simulink library "UXFD_Lib"  (R2016b)
settings: Solver=ode45  StartTime=0.0  StopTime=10.0  RelTol=1e-3  EnableMultiTasking=on
undefined symbols (not defined in the file): BreakpointData, BreakpointData1, BreakpointData2, BreakpointData_One_A, BreakpointData_Two_A, E2E_P01DataIDMode, E2E_P01ReceiverStatusType, EnumClass, iBit, initalValue, No_Runnable_Period, ObB_EidBsgStDerat_C, p_OVERRIDE_MASTER_SWITCH, SlDemoSign, SwitchOff_P, SwitchOn_P, Table, TableData_M, VCCTi33, VSysD_FidVehDerat1_C
libraries: simulink x28, CCMLib x11, UXFD_Lib x8, canmsglib x2, PTCC_Lib x1, hdlsllib x1
(part 3 of 7)

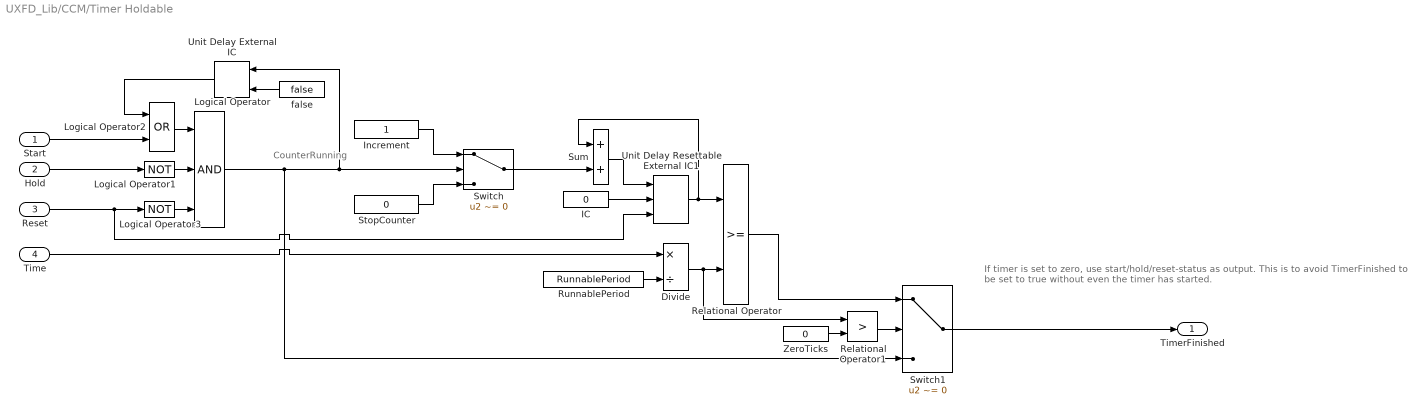
== system UXFD_Lib/CCM/Timer Holdable ==
  note: If timer is set to zero, use start/hold/reset-status as output.
      | This is to avoid TimerFinished to be set to true without even the timer has started.
  note: CounterRunning
  Start : Inport  OutDataTypeStr=boolean
  Hold : Inport  Port=2  OutDataTypeStr=boolean
  Reset : Inport  Port=3  OutDataTypeStr=boolean
  Time : Inport  Port=4  OutDataTypeStr=timeDataType
  Divide : Product  Inputs=*/  OutDataTypeStr=VCCUInt32  RndMeth=Round  SaturateOnIntegerOverflow=on
  IC : Constant  Value=0  OutDataTypeStr=VCCUInt32  SampleTime=-1
  Increment : Constant  OutDataTypeStr=VCCUInt32  SampleTime=-1
  Logical Operator : Logic  Inputs=3  AllPortsSameDT=off  OutDataTypeStr=boolean
  Logical Operator1 : Logic  Operator=NOT  AllPortsSameDT=off  OutDataTypeStr=boolean
  Logical Operator2 : Logic  Operator=OR  AllPortsSameDT=off  OutDataTypeStr=boolean
  Logical Operator3 : Logic  Operator=NOT  AllPortsSameDT=off  OutDataTypeStr=boolean
  Relational Operator : RelationalOperator  OutDataTypeStr=boolean  RndMeth=Nearest
  Relational Operator1 : RelationalOperator  Operator=>  OutDataTypeStr=boolean  RndMeth=Nearest
  RunnablePeriod : Constant  Value=RunnablePeriod  OutDataTypeStr=VCCTiSamplePerd  SampleTime=-1
  StopCounter : Constant  Value=0  OutDataTypeStr=VCCUInt32  SampleTime=-1
  Sum : Sum  OutDataTypeStr=VCCUInt32  SaturateOnIntegerOverflow=on
  Switch : Switch  Criteria=u2 ~= 0  SaturateOnIntegerOverflow=on
  Switch1 : Switch  Criteria=u2 ~= 0  SaturateOnIntegerOverflow=on
  Unit Delay External IC : simulink/Additional Math & Discrete/Additional Discrete/Unit Delay External IC  tsamp=-1
  Unit Delay Resettable External IC1 : CCMLib/Unit Delay Resettable External IC  dataType=VCCUInt32
  ZeroTicks : Constant  Value=0  OutDataTypeStr=VCCUInt32  SampleTime=-1
  false : Constant  Value=false  OutDataTypeStr=boolean  SampleTime=-1
  TimerFinished : Outport  OutDataTypeStr=boolean
  wires:
  Sum/1 -> Unit Delay Resettable External IC1/1
  IC/1 -> Unit Delay Resettable External IC1/2
  Time/1 -> Divide/1
  Reset/1 -> Unit Delay Resettable External IC1/3, Logical Operator3/1
  Logical Operator3/1 -> Logical Operator/3
  Switch1/1 -> TimerFinished/1
  Divide/1 -> Relational Operator1/1, Relational Operator/2
  Relational Operator/1 -> Switch1/1
  Relational Operator1/1 -> Switch1/2
  ZeroTicks/1 -> Relational Operator1/2
  RunnablePeriod/1 -> Divide/2
  StopCounter/1 -> Switch/3
  Increment/1 -> Switch/1
  Switch/1 -> Sum/2
  Unit Delay Resettable External IC1/1 -> Relational Operator/1, Sum/1
  Unit Delay External IC/1 -> Logical Operator2/1
  Start/1 -> Logical Operator2/2
  Logical Operator/1 -> Switch1/3, Unit Delay External IC/1, Switch/2
  false/1 -> Unit Delay External IC/2
  Logical Operator2/1 -> Logical Operator/1
  Hold/1 -> Logical Operator1/1
  Logical Operator1/1 -> Logical Operator/2

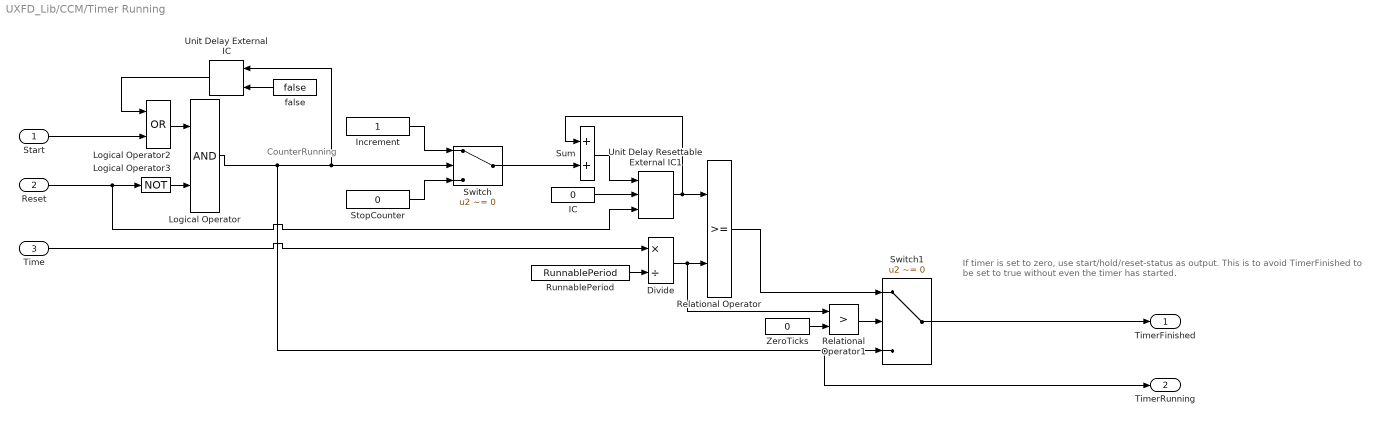
== system UXFD_Lib/CCM/Timer Running ==
  note: If timer is set to zero, use start/hold/reset-status as output.
      | This is to avoid TimerFinished to be set to true without even the timer has started.
  note: CounterRunning
  Start : Inport  OutDataTypeStr=boolean
  Reset : Inport  Port=2  OutDataTypeStr=boolean
  Time : Inport  Port=3  OutDataTypeStr=timeDataType
  Divide : Product  Inputs=*/  OutDataTypeStr=VCCUInt32  RndMeth=Round  SaturateOnIntegerOverflow=on
  IC : Constant  Value=0  OutDataTypeStr=VCCUInt32  SampleTime=-1
  Increment : Constant  OutDataTypeStr=VCCUInt32  SampleTime=-1
  Logical Operator : Logic  AllPortsSameDT=off  OutDataTypeStr=boolean
  Logical Operator2 : Logic  Operator=OR  AllPortsSameDT=off  OutDataTypeStr=boolean
  Logical Operator3 : Logic  Operator=NOT  AllPortsSameDT=off  OutDataTypeStr=boolean
  Relational Operator : RelationalOperator  OutDataTypeStr=boolean  RndMeth=Nearest
  Relational Operator1 : RelationalOperator  Operator=>  OutDataTypeStr=boolean  RndMeth=Nearest
  RunnablePeriod : Constant  Value=RunnablePeriod  OutDataTypeStr=VCCTiSamplePerd  SampleTime=-1
  StopCounter : Constant  Value=0  OutDataTypeStr=VCCUInt32  SampleTime=-1
  Sum : Sum  OutDataTypeStr=VCCUInt32  SaturateOnIntegerOverflow=on
  Switch : Switch  Criteria=u2 ~= 0  SaturateOnIntegerOverflow=on
  Switch1 : Switch  Criteria=u2 ~= 0  SaturateOnIntegerOverflow=on
  Unit Delay External IC : simulink/Additional Math & Discrete/Additional Discrete/Unit Delay External IC  tsamp=-1
  Unit Delay Resettable External IC1 : CCMLib/Unit Delay Resettable External IC  dataType=VCCUInt32
  ZeroTicks : Constant  Value=0  OutDataTypeStr=VCCUInt32  SampleTime=-1
  false : Constant  Value=false  OutDataTypeStr=boolean  SampleTime=-1
  TimerFinished : Outport  OutDataTypeStr=boolean
  TimerRunning : Outport  Port=2  OutDataTypeStr=boolean
  wires:
  Sum/1 -> Unit Delay Resettable External IC1/1
  IC/1 -> Unit Delay Resettable External IC1/2
  Time/1 -> Divide/1
  Reset/1 -> Unit Delay Resettable External IC1/3, Logical Operator3/1
  Logical Operator3/1 -> Logical Operator/2
  Switch1/1 -> TimerFinished/1
  Divide/1 -> Relational Operator1/1, Relational Operator/2
  Relational Operator/1 -> Switch1/1
  Relational Operator1/1 -> Switch1/2
  ZeroTicks/1 -> Relational Operator1/2
  RunnablePeriod/1 -> Divide/2
  StopCounter/1 -> Switch/3
  Increment/1 -> Switch/1
  Switch/1 -> Sum/2
  Unit Delay Resettable External IC1/1 -> Sum/1, Relational Operator/1
  Unit Delay External IC/1 -> Logical Operator2/1
  Start/1 -> Logical Operator2/2
  Logical Operator/1 -> TimerRunning/1, Switch1/3, Unit Delay External IC/1, Switch/2
  false/1 -> Unit Delay External IC/2
  Logical Operator2/1 -> Logical Operator/1

== system UXFD_Lib/CCM/Unit Delay External IC ==
  u : Inport  OutDataTypeStr=dataType
  IC : Inport  Port=2  OutDataTypeStr=dataType
  Constant : Constant  Value=true  OutDataTypeStr=boolean  SampleTime=-1
  Switch : Switch  Criteria=u2 ~= 0  SaturateOnIntegerOverflow=on
  Unit Delay : UnitDelay  InitialCondition=false  SampleTime=-1
      settings: AttributesFormatString=X0=%<X0>
  Unit Delay1 : UnitDelay  SampleTime=-1
      settings: AttributesFormatString=X0=%<X0>
  y : Outport  OutDataTypeStr=dataType
  wires:
  Switch/1 -> y/1
  IC/1 -> Switch/3
  u/1 -> Unit Delay1/1
  Unit Delay1/1 -> Switch/1
  Constant/1 -> Unit Delay/1
  Unit Delay/1 -> Switch/2

== system UXFD_Lib/CCM/Unit Delay Resettable ==
  u : Inport  OutDataTypeStr=dataType
  R : Inport  Port=2  OutDataTypeStr=boolean
  Constant : Constant  Value=false  OutDataTypeStr=boolean  SampleTime=-1
  Logical Operator : Logic  Operator=OR  AllPortsSameDT=off  OutDataTypeStr=boolean
  Logical Operator1 : Logic  Operator=NOT  AllPortsSameDT=off  OutDataTypeStr=boolean
  Switch : Switch  Criteria=u2 ~= 0  SaturateOnIntegerOverflow=on
  Switch1 : Switch  Criteria=u2 ~= 0  SaturateOnIntegerOverflow=on
  Unit Delay : UnitDelay  InitialCondition=true  SampleTime=-1
      settings: AttributesFormatString=X0=%<X0>
  Unit Delay1 : UnitDelay  InitialCondition=initialCondition  SampleTime=-1
      settings: AttributesFormatString=X0=%<X0>
  initialCondition : Constant  Value=initialCondition  OutDataTypeStr=dataType  SampleTime=-1
  y : Outport  OutDataTypeStr=dataType
  wires:
  Constant/1 -> Unit Delay/1
  Switch/1 -> y/1
  Logical Operator/1 -> Switch/2
  Unit Delay/1 -> Logical Operator/2
  R/1 -> Logical Operator/1, Logical Operator1/1
  Logical Operator1/1 -> Switch1/2
  initialCondition/1 -> Switch1/3, Switch/1
  Switch1/1 -> Unit Delay1/1
  Unit Delay1/1 -> Switch/3
  u/1 -> Switch1/1

== system UXFD_Lib/CCM/Unit Delay Resettable External IC ==
  u : Inport  OutDataTypeStr=dataType
  IC : Inport  Port=2  OutDataTypeStr=dataType
  R : Inport  Port=3  OutDataTypeStr=boolean
  Constant : Constant  Value=true  OutDataTypeStr=boolean  SampleTime=-1
  Logical Operator : Logic  Operator=NOT  AllPortsSameDT=off  OutDataTypeStr=boolean
  Logical Operator1 : Logic  AllPortsSameDT=off  OutDataTypeStr=boolean
  Switch : Switch  Criteria=u2 ~= 0  SaturateOnIntegerOverflow=on
  Switch1 : Switch  Criteria=u2 ~= 0  SaturateOnIntegerOverflow=on
  Unit Delay : UnitDelay  InitialCondition=false  SampleTime=-1
      settings: AttributesFormatString=X0=%<X0>
  Unit Delay1 : UnitDelay  SampleTime=-1
      settings: AttributesFormatString=X0=%<X0>
  y : Outport  OutDataTypeStr=dataType
  wires:
  Logical Operator1/1 -> Switch/2
  Unit Delay/1 -> Logical Operator1/1
  Switch1/1 -> Unit Delay1/1
  IC/1 -> Switch/3, Switch1/3
  u/1 -> Switch1/1
  R/1 -> Logical Operator/1
  Logical Operator/1 -> Logical Operator1/2, Switch1/2
  Constant/1 -> Unit Delay/1
  Unit Delay1/1 -> Switch/1
  Switch/1 -> y/1

== system UXFD_Lib/Custom/CAN ==
  note: CAN
  CAN Pack : canmsglib/CAN Pack  MsgList=(none)  MsgName=CAN Msg  MsgIDType=Standard (11-bit identifier)  MsgIdentifier=0  MsgLength=8  NSignals=0  StartBits=0  SignalSizes=0  ByteOrders=0  DataTypes=0  MultiplexTypes=0  MultiplexValues=0  Factors=0  Offsets=0  Minimums=0  Maximums=0  Remote=off
      settings: DataFormat=raw data
  CAN Unpack : canmsglib/CAN Unpack  MsgName=CAN Msg  MsgIDType=Standard (11-bit identifier)  MsgIdentifier=0  MsgLength=8  NSignals=0  IDPort=off  TimestampPort=off  ErrorPort=off  RemotePort=off  LengthPort=off  StatusPort=off  StartBits=0  SignalSizes=0  ByteOrders=0  DataTypes=0  MultiplexTypes=0  MultiplexValues=0  Factors=0  Offsets=0  Minimums=0  Maximums=0
      settings: DataFormat=raw data
  CAN_Receive : Subsystem  mask(CAN Message Receive( GLib TM )){}
      mask help:
      | Input： DataType CAN_Message Signal and handle
      | Output：If Received success , Return Value is 1
      mask Display:
      | port_label('input',1,'Message')
      | port_label('input',2,'Handle')
      | port_label('output',1,'ReturnValue')
      | disp('ACTION_CANBSW_RecMsg_S')
  CAN_Transmit : Subsystem  mask(CAN Message Transmit( GLib TM )){}
      mask help:
      | Input： DataType CAN_Message Signal and handle
      | Output：If Transmited success , Return Value is 1
      mask Display:
      | port_label('input',1,'Message')
      | port_label('input',2,'Handle')
      | port_label('output',1,'ReturnValue')
      | disp('ACTION_CANBSW_SndMsg_S')
  CanHex2Signed : Subsystem  mask(CAN signal Hex2Signed){BitLengthValue=32, FactorValue=0.001, OffsetValue=0}
      mask prompts: BitLengthValue "CAN Signal Bit Length（0<u<=32bit）"; FactorValue "Factor"; OffsetValue "Offset"
      mask help: convert the hex to signed value, please specified bit length of varible in CAN matrix, the maximum bit length in CAN matrixa may be 32bit; Also, please specified the factor and offset, then execute Phy=hex*factor+offset.
      mask init:
      | % The mask parameter returns the one-based index of the selection
      | FactorValue;
      | OffsetValue;
      | BitLengthValue;
      | % To obtain the string corresponding to the selection, use get_param
      | blk = gcb;
      | FactorString = get_param(blk,'FactorValue');
      | OffsetString = get_param(blk,'OffsetValue');
      | BitSzieString = get_param(blk,'BitLengthValue');
      | 
      |     % Convert the string into a single to use the value under the mask
      |     BitLength = single(str2num(BitSzieString)); 
      |     Factor=single(str2num(FactorString)); 
      |     Offset=single(str2num(OffsetString));
      mask Display:
      | fprintf('CAN signal convert\nBitLength: %d\nFactor: %2.4f\nOffset: %2.4f',...
      |     BitLengthValue,FactorValue,OffsetValue);
  Get_MsgLength : Subsystem  mask(Get CAN Message Length( GLib TM )){}
      mask help:
      | Input： DataType CAN_Message Signal
      | Output：CAN Message Length
      mask Display:
      | port_label('input',1,'Message')
      | port_label('output',1,'Length')
      | disp('Msg_Length_S')
  xbackground1 : Subsystem
      mask Display: disp(' ')

== system UXFD_Lib/Custom/Diagnose ==
  note: Diagnose
  Dem_SetEventStatus : Subsystem  mask(SL Blockset Dem_SetEventStatus){EventID=ObB_EidBsgStDerat_C}
      mask prompts: EventID "Dem Event ID"
      mask help:
      | Interface block to call Dem_SetEventStatus.
      | The output of the block can be captured by using Dem_SetEventStatus blocks with the same EventID.
      mask TypeOptions EventID: DEM_EventID/Value
      mask Display:
      | id = get_param(gcb,'EventID');
      | text(0.55,0.9,sprintf('Dem_SetEventStatus\nEventID: %s', id),...
      |     'horizontalAlignment','center',...
      |     'verticalAlignment', 'top');
      | 
      | 
      | port_label('input',1,'EveSt');
      | port_label('input',2,'bEna');
  Fim_GetFunctionPermission : Subsystem  mask(SL Blockset Fim_GetFunctionPermission){FunctionID=VSysD_FidVehDerat1_C}
      mask prompts: FunctionID "FIM FunctionID"
      mask help:
      | Interface block to call Fim_GetFunctionPermission.
      | The output of the block can be stimulated by using Fim_GetFunctionPermission_Stimuli blocks with the same FunctionID.
      mask TypeOptions FunctionID: FIM_EventID/Value
      mask Display:
      | id = get_param(gcb,'FunctionID');
      | text(0.45,0.9,sprintf('Fim_GetFunctionPermission\nFunctionID: %s', id),...
      |     'horizontalAlignment','center',...
      |     'verticalAlignment', 'top');
      | 
      | port_label('output',1,'bEna');
  xbackground1 : Subsystem
      mask Display: disp(' ')

== system UXFD_Lib/Custom/PIN ==
  note: HW PIN
  PIN ADC : Subsystem  mask(PIN ADC){g_functionName=Sws_Io_Adc_Get_xxx, g_getValue=2}
      mask prompts: g_functionName "应用层接口函数"; g_getValue "测试输出返回值"
      mask help:
      | This block is for ASW to get Hardware's  ADC PIN Value
      | Function: uint16 Sws_Io_Adc_Get_xxx(void)
      mask Display: text(0.08,0.67,'Get Pin Analog Input','horizontalAlignment', 'left', 'verticalAlignment', 'top');
  PIN DI : Subsystem  mask(PIN DI){g_functionName=Sws_Io_Dio_Get_xxx, g_getValue=1}
      mask prompts: g_functionName "应用层接口函数"; g_getValue "测试输出返回值"
      mask help:
      | This block is for ASW to get Hardware's  DI PIN Value
      | Function: boolean Sws_Io_Dio_Get_xxx()
      mask Display: text(0.08,0.67,'Get Pin Digital Input','horizontalAlignment', 'left', 'verticalAlignment', 'top');
  PIN DO : Subsystem  mask(PIN DO){g_functionName=Sws_Io_Dio_Set_O_S_xxx}
      mask prompts: g_functionName "应用层接口函数"
      mask help:
      | This block is for ASW to set Hardware's  DO PIN Value
      | Function:  void Sws_Io_Dio_Set_O_S_xxx(boolean stSignal_b)
      mask Display: text(0.08,0.67,'Set Pin Digital Output','horizontalAlignment', 'left', 'verticalAlignment', 'top');
  PIN DO1 : Subsystem  mask(PIN PWMOUT){g_functionName=Sws_Io_PWM_Set_O_S_xxx}
      mask prompts: g_functionName "应用层接口函数"
      mask help:
      | This block is for ASW to set Hardware's  PWM PIN Value
      | Function:  void Sws_Io_PWM_Set_O_S_xxx(sint16 Duty_s16,uint32 Period_u32)
      mask Display: text(0.08,0.67,'Set Pin PWM Output','horizontalAlignment', 'left', 'verticalAlignment', 'top');
  PIN ICU : Subsystem  mask(PIN ICU){g_functionName=Sws_Io_Icu_GetPeriod_xxx, g_getValue=50}
      mask prompts: g_functionName "应用层接口函数"; g_getValue "测试输出返回值"
      mask help:
      | This block is for ASW to get Hardware's  ICU PIN Value
      | Function:  Sws_Io_Icu_GetDutyCyclexxx(void)
      mask Display: text(0.08,0.67,'Get Pin ICU Input','horizontalAlignment', 'left', 'verticalAlignment', 'top');
  xbackground1 : Subsystem
      mask Display: disp(' ')

== system UXFD_Lib/Standard/Bit Operation ==
  Bit Clear : simulink/Logic and Bit Operations/Bit Clear  iBit=0
  Bit Set : simulink/Logic and Bit Operations/Bit Set  iBit=0
  Bit Shift : hdlsllib/HDL Operations/Bit Shift  mode=Shift Left Logical  N=0
  Bitwise OR : simulink/Logic and Bit Operations/Bitwise Operator  logicop=OR  UseBitMask=off  BitMask=2.^iBit  BitMaskRealWorld=Stored Integer
  Bitwise Operator : simulink/Logic and Bit Operations/Bitwise Operator  logicop=AND  UseBitMask=on  BitMask=bin2dec('11011001')  BitMaskRealWorld=Stored Integer
  GetBitFnc : Subsystem  mask(Bit Get){GetBitPar=2, U8Par=uint32, BitMinPar=0, BitMaxPar=31}
      mask prompts: GetBitPar "GetBit"; U8Par "DataTypeSelect"; BitMinPar "BitMin"; BitMaxPar "BitMax"
      mask help: Input bit value, then select the bit position you want
      settings: CopyFcn=set_param(gcb, 'LinkStatus', 'none');
      mask Callback GetBitPar:
      | if isequal(get_param(gcb,'U8Par'),'uint8')
      |     set_param(gcb,'BitMinPar','0');
      |     set_param(gcb,'BitMaxPar','7');
      |     if str2double(get_param(gcb,'GetBitPar')) > 7
      |         set_param(gcb,'GetBitPar','7');
      |     elseif str2double(get_param(gcb,'GetBitPar')) < 0
      |         set_param(gcb,'GetBitPar','0');
      |     else
      |         set_param(gcb,'GetBitPar',num2str(uint8(str2double(get_param(gcb,'GetBitPar')))));
      |     end
      | elseif isequal(get_param(gcb,'U8Par'),'uint16')
      |     set_param(gcb,'BitMinPar','0');
      |     set_param(gcb,'BitMaxPar','15');
      |     if str2double(get_param(gcb,'GetBitPar')) > 15
      |         set_param(gcb,'GetBitPar','15');
      |     elseif str2double(get_param(gcb,'GetBitPar')) < 0
      |         set_param(gcb,'GetBitPar','0');
      |     else
      |         set_param(gcb,'GetBitPar',num2str(uint16(str2double(get_param(gcb,'GetBitPar')))));
      |     end
      | else
      |     set_param(gcb,'BitMinPar','0');
      |     set_param(gcb,'BitMaxPar','31');
      |     if str2double(get_param(gcb,'GetBitPar')) > 31
      |         set_param(gcb,'GetBitPar','31');
      |     elseif str2double(get_param(gcb,'GetBitPar')) < 0
      |         set_param(gcb,'GetBitPar','0');
      |     else
      |         set_param(gcb,'GetBitPar',num2str(uint32(str2double(get_param(gcb,'GetBitPar')))));
      |     end
      | end
      | set_param([gcb '/Getbit_n'],'value',['uint8(' get_param(gcb,'GetBitPar') ')']);
      mask TypeOptions U8Par: uint8 | uint16 | uint32
      mask Callback U8Par:
      | if isequal(get_param(gcb,'U8Par'),'uint8')
      |     set_param(gcb,'BitMinPar','0');
      |     set_param(gcb,'BitMaxPar','7');
      |     if str2double(get_param(gcb,'GetBitPar')) > 7
      |         set_param(gcb,'GetBitPar','7');
      |     elseif str2double(get_param(gcb,'GetBitPar')) < 0
      |         set_param(gcb,'GetBitPar','0');
      |     end
      | %     set_param([gcb '/BitWise'],'BitMask',['bin2dec(' '''' '11111111' '''' ')']);
      |     set_param([gcb '/Min'],'value','uint8(0)');
      |     set_param([gcb '/Max'],'value','uint8(7)');
      |     set_param([gcb '/BitVal'],'OutDataTypeStr','uint8');
      | elseif isequal(get_param(gcb,'U8Par'),'uint16')
      |     set_param(gcb,'BitMinPar','0');
      |     set_param(gcb,'BitMaxPar','15');
      |     if str2double(get_param(gcb,'GetBitPar')) > 15
      |         set_param(gcb,'GetBitPar','15');
      |     elseif str2double(get_param(gcb,'GetBitPar')) < 0
      |         set_param(gcb,'GetBitPar','0');
      |     end
      | %     set_param([gcb '/BitWise'],'BitMask',['bin2dec(' '''' '1111111111111111' '''' ')']);
      |     set_param([gcb '/Min'],'value','uint8(0)');
      |     set_param([gcb '/Max'],'value','uint8(15)');
      |     set_param([gcb '/BitVal'],'OutDataTypeStr','uint16');
      | else
      |     set_param(gcb,'BitMinPar','0');
      |     set_param(gcb,'BitMaxPar','31');
      |     if str2double(get_param(gcb,'GetBitPar')) > 31
      |         set_param(gcb,'GetBitPar','31');
      |     elseif str2double(get_param(gcb,'GetBitPar')) < 0
      |         set_param(gcb,'GetBitPar','0');
      |     end
      | %     set_param([gcb '/BitWise'],'BitMask',['bin2dec(' '''' '11111111111111111111111111111111' '''' ')']);
      |     set_param([gcb '/Min'],'value','uint8(0)');
      |     set_param([gcb '/Max'],'value','uint8(31)');
      |     set_param([gcb '/BitVal'],'OutDataTypeStr','uint32');
      | end
      mask Display:
      | % disp(dispStr)
      | % id = get_param(gcb,'GetBitPar');
      | % text(0.55,0.9,sprintf('Getbit_Uint8\n', id),...
      | %     'horizontalAlignment','center',...
      | %     'verticalAlignment', 'top');
      | disp([GetBitPar]);
      | port_label('input', 1, 'BitVal_B');
      | port_label('output', 1, 'Val');
  SetBitFnc : Subsystem  mask(Bit Set){SetBitPar=5, U8Par=uint32, BitMinPar=0, BitMaxPar=31}
      mask prompts: SetBitPar "SetBit"; U8Par "DataTypeSelect"; BitMinPar "BitMin"; BitMaxPar "BitMax"
      mask help: Input bit value, then select the bit position you want
      mask Callback SetBitPar:
      | if isequal(get_param(gcb,'U8Par'),'uint8')
      |     set_param(gcb,'BitMinPar','0');
      |     set_param(gcb,'BitMaxPar','7');
      |     if str2double(get_param(gcb,'SetBitPar')) > 7
      |         set_param(gcb,'SetBitPar','7');
      |     elseif str2double(get_param(gcb,'SetBitPar')) < 0
      |         set_param(gcb,'SetBitPar','0');
      |     else
      |         set_param(gcb,'SetBitPar',num2str(uint8(str2double(get_param(gcb,'SetBitPar')))));
      |     end
      | elseif isequal(get_param(gcb,'U8Par'),'uint16')
      |     set_param(gcb,'BitMinPar','0');
      |     set_param(gcb,'BitMaxPar','15');
      |     if str2double(get_param(gcb,'SetBitPar')) > 15
      |         set_param(gcb,'SetBitPar','15');
      |     elseif str2double(get_param(gcb,'SetBitPar')) < 0
      |         set_param(gcb,'SetBitPar','0');
      |     else
      |         set_param(gcb,'SetBitPar',num2str(uint16(str2double(get_param(gcb,'SetBitPar')))));
      |     end
      | else
      |     set_param(gcb,'BitMinPar','0');
      |     set_param(gcb,'BitMaxPar','31');
      |     if str2double(get_param(gcb,'SetBitPar')) > 31
      |         set_param(gcb,'SetBitPar','31');
      |     elseif str2double(get_param(gcb,'SetBitPar')) < 0
      |         set_param(gcb,'SetBitPar','0');
      |     else
      |         set_param(gcb,'SetBitPar',num2str(uint32(str2double(get_param(gcb,'SetBitPar')))));
      |     end
      | end
      | set_param([gcb '/Setbit_n'],'value',['uint8(' get_param(gcb,'SetBitPar') ')']);
      mask TypeOptions U8Par: uint8 | uint16 | uint32
      mask Callback U8Par:
      | if isequal(get_param(gcb,'U8Par'),'uint8')
      |     set_param(gcb,'BitMinPar','0');
      |     set_param(gcb,'BitMaxPar','7');
      |     if str2double(get_param(gcb,'SetBitPar')) > 7
      |         set_param(gcb,'SetBitPar','7');
      |     elseif str2double(get_param(gcb,'SetBitPar')) < 0
      |         set_param(gcb,'SetBitPar','0');
      |     end
      |     set_param([gcb '/BitWise'],'BitMask',['bin2dec(' '''' '11111111' '''' ')']);
      |     set_param([gcb '/Min'],'value','uint8(0)');
      |     set_param([gcb '/Max'],'value','uint8(7)');
      |     set_param([gcb '/Product'],'OutDataTypeStr','uint8');
      | elseif isequal(get_param(gcb,'U8Par'),'uint16')
      |     set_param(gcb,'BitMinPar','0');
      |     set_param(gcb,'BitMaxPar','15');
      |     if str2double(get_param(gcb,'SetBitPar')) > 15
      |         set_param(gcb,'SetBitPar','15');
      |     elseif str2double(get_param(gcb,'SetBitPar')) < 0
      |         set_param(gcb,'SetBitPar','0');
      |     end
      |     set_param([gcb '/BitWise'],'BitMask',['bin2dec(' '''' '1111111111111111' '''' ')']);
      |     set_param([gcb '/Min'],'value','uint8(0)');
      |     set_param([gcb '/Max'],'value','uint8(15)');
      |     set_param([gcb '/Product'],'OutDataTypeStr','uint16');
      | else
      |     set_param(gcb,'BitMinPar','0');
      |     set_param(gcb,'BitMaxPar','31');
      |     if str2double(get_param(gcb,'SetBitPar')) > 31
      |         set_param(gcb,'SetBitPar','31');
      |     elseif str2double(get_param(gcb,'SetBitPar')) < 0
      |         set_param(gcb,'SetBitPar','0');
      |     end
      |     set_param([gcb '/BitWise'],'BitMask',['bin2dec(' '''' '11111111111111111111111111111111' '''' ')']);
      |     set_param([gcb '/Min'],'value','uint8(0)');
      |     set_param([gcb '/Max'],'value','uint8(31)');
      |     set_param([gcb '/Product'],'OutDataTypeStr','uint32');
      | end
      mask Display:
      | disp([SetBitPar]);
      | port_label('input', 1, 'BitVal_B');
      | port_label('output', 1, 'Val');
  Shift Arithmetic : ArithShift  BitShiftNumber=8
      settings: CopyFcn=set_param(gcbh,'ShowName','off');
  xbackground4 : UXFD_Lib/xbackground4  SystemSampleTime=-1

== system UXFD_Lib/Standard/Calibration ==
  note: Look-up masks including
      | lookup and prelookup blocks
  note: Look-up and pre-lookup blocks
  note: Calibration
  note: OverRide
  1-D Lookup Table : Lookup  InputValues=BreakpointData  Table=Table  LookUpMeth=Interpolation-Use End Values  OutDataTypeStr=single
      settings: CopyFcn=set_param(gcbh,'ShowName','on');
  1-D Lookup Table Without Const_Param : Subsystem  Tag=AVLib calibration  mask(Lookup Table 1D){BlockConfiguration=freeze, BreakpointData=BreakpointData, ReferenceBreakpointData=off, OpenMPTBreakpointData=off, OpenADDBreakpointData=off, IndexSearchMethod=Linear search, Table=Table, ReferenceTable=off, OpenMPTTable=off, OpenADDTable=off, InterpMethod=Linear, DisplayCalibrationNames=off, AdoptBlockName=off, OutMin=[], OutMax=[], OutDataType=Inherit: Inherit from data, IndexDataType=uint8, FractionDataType=Inherit: Inherit via internal rule}
      mask prompts: BlockConfiguration "Block configuration:"; BreakpointData "Breakpoint data:"; ReferenceBreakpointData "Treat as calibration reference"; OpenMPTBreakpointData "Open breakpoint data"; OpenADDBreakpointData "Open ADD breakpoint data"; IndexSearchMethod "Index search method:"; Table "Table data:"; ReferenceTable "Treat as calibration reference"; OpenMPTTable "Open table data"; OpenADDTable "Open ADD table data"; InterpMethod "Interpolation method:"; DisplayCalibrationNames "Block annotation with calibration data"; AdoptBlockName "Adopt block name from table name"; OutMin "Output minimum:"; OutMax "Output maximum:"; OutDataType "Output data type:"; IndexDataType "Index data type:"; FractionDataType "Fraction data type:"
      mask help: Perform 1-D linear interpolation of input values using the specified table.
      mask init:
      | % get and transmit data type from value
      | if strcmp(OutDataType,'Inherit: Inherit from data')
      |   val = Table;  nam = get_param(gcb,'Table');
      |   if evalin('base',['exist(''',nam,''',''var'')']),  s = evalin('base',nam);
      |     if isa(s,'mpt.Parameter') || isa(s,'Simulink.Parameter') || isa(s,'AVLmpt.Parameter')
      |       valDataType = s.DataType;
      |       if strcmp(valDataType,'auto'), valDataType = 'double'; end
      |     else
      |       valDataType = class(s);
      |     end
      |   else
      |       valDataType = class(val);
      |   end
      |   if strcmp(valDataType,'logical'), valDataType = 'boolean'; end
      |   set_param([gcb,'/Curve'],'OutDataTypeStr',valDataType)
      | end
      | if 1
      |   val = BreakpointData;  nam = get_param(gcb,'BreakpointData');
      |   if evalin('base',['exist(''',nam,''',''var'')']),  s = evalin('base',nam);
      |     if isa(s,'mpt.Parameter') || isa(s,'Simulink.Parameter') || isa(s,'AVLmpt.Parameter')
      |       valDataType = s.DataType;
      |       if strcmp(valDataType,'auto'), valDataType = 'double'; end
      |     else
      |       valDataType = class(s);
      |     end
      |   else
      |       valDataType = class(val);
      |   end
      |   if strcmp(valDataType,'logical'), valDataType = 'boolean'; end
      |   set_param([gcb,'/u'],'OutDataTypeStr',valDataType)
      | end
      | 
      | % © AVL S&F, C.A. Roduner, Nov/18/2009
      | if BlockConfiguration==1 && (~strcmp(get_param(gcb,'LinkStatus'),'resolved') ...
      |   || (~strncmp(get_param(gcb,'Referenceblock'),'AVLib',5) && ~exist('AVLib_Init','file') ) ), return, end
      | AVLib_Init( 'LookupTable1D_init', gcb, ...
      |   BlockConfiguration,IndexSearchMethod,InterpMethod, ...
      |   DisplayCalibrationNames,AdoptBlockName,  ...
      |   BreakpointData,ReferenceBreakpointData,OpenMPTBreakpointData, OpenADDBreakpointData, ...
      |   Table,ReferenceTable,OpenMPTTable,OpenADDTable, ...
      |   IndexDataType, FractionDataType, ...
      |   OutMin,OutMax,OutDataType ...
      | );
      mask Help: eval('try openDocu(gcb), catch try run([fileparts(which(''AVLib'')),''\..\AVLibDocu\openDocu'']), catch errordlg(''No documentation available on Matlab path.'',gcb,''modal''), end, end')
      mask TypeOptions BlockConfiguration: freeze | enable | default
      mask Callback BreakpointData:
      | if strcmp(get_param(gcb,'BlockConfiguration'),'freeze'), return, end
      | AVLib_Init('Calibration_cb',gcb,'BreakpointData')
      mask Callback OpenMPTBreakpointData:
      | if strcmp(get_param(gcb,'BlockConfiguration'),'freeze'), return, end
      | AVLib_Init('OpenMPT_cb',gcb,'BreakpointData')
      mask Callback OpenADDBreakpointData:
      | if strcmp(get_param(gcb,'BlockConfiguration'),'freeze'), return, end
      | if strcmp(get_param(gcb,'OpenADDBreakpointData'),'on')
      |   set_param(gcb,'OpenADDBreakpointData','off')
      |   set_param(gcb,'BreakpointData', connectADD(get_param(gcb,'BreakpointData'),'axis') )
      | end
      mask TypeOptions IndexSearchMethod: Evenly spaced points | Linear search | Binary search
      mask Callback Table:
      | if strcmp(get_param(gcb,'BlockConfiguration'),'freeze'), return, end
      | AVLib_Init('Calibration_cb',gcb,'Table')
      mask Callback OpenMPTTable:
      | if strcmp(get_param(gcb,'BlockConfiguration'),'freeze'), return, end
      | AVLib_Init('OpenMPT_cb',gcb,'Table')
      mask Callback OpenADDTable:
      | if strcmp(get_param(gcb,'BlockConfiguration'),'freeze'), return, end
      | if strcmp(get_param(gcb,'OpenADDTable'),'on')
      |   set_param(gcb,'OpenADDTable','off')
      |   set_param(gcb,'Table', connectADD(get_param(gcb,'Table'),'curve') )
      | end
      mask TypeOptions InterpMethod: None - Flat | Linear
      mask Callback AdoptBlockName:
      | if strcmp(get_param(gcb,'BlockConfiguration'),'freeze'), return, end
      | AVLib_Init('AdoptBlockName_cb',gcb,get_param(gcb,'Table'))
      mask TypeOptions OutDataType: Inherit: Inherit from data | Inherit: Inherit via back propagation | double | single | int8 | uint8 | int16 | uint16 | int32 | uint32 | boolean
      mask TypeOptions IndexDataType: uint8 | uint16 | uint32
      mask TypeOptions FractionDataType: Inherit: Inherit via internal rule | double | single
      mask Display:
      | plot( getfield(get_param(gcb,'UserData'),'xy') )
      | plot( getfield(get_param(gcb,'UserData'),'xy_InterpMethod') )
      | color('blue'), plot( getfield(get_param(gcb,'UserData'),'xy_C') )
  2-D Lookup Table : Lookup2D  RowIndex=BreakpointData1  ColumnIndex=BreakpointData2  Table=Table  LookUpMeth=Interpolation-Use End Values  OutDataTypeStr=single
      settings: CopyFcn=set_param(gcbh,'ShowName','on');
  2-D Lookup Table Without Const_Param : Subsystem  Tag=AVLib calibration  mask(Lookup Table 2D){BlockConfiguration=freeze, BreakpointData1=BreakpointData1, ReferenceBreakpointData1=off, OpenMPTBreakpointData1=off, OpenADDBreakpointData1=off, BreakpointData2=BreakpointData2, ReferenceBreakpointData2=off, OpenMPTBreakpointData2=off, OpenADDBreakpointData2=off, IndexSearchMethod=Binary search, Table=Table, ReferenceTable=off, OpenMPTTable=off, OpenADDTable=off, InterpMethod=Linear, DisplayCalibrationNames=off, AdoptBlockName=off, OutMin=[], OutMax=[], OutDataType=Inherit: Inherit from data, IndexDataType=uint8, FractionDataType=Inherit: Inherit via internal rule}
      mask prompts: BlockConfiguration "Block configuration:"; BreakpointData1 "Breakpoint data for 1st input (x-axis, row index):"; ReferenceBreakpointData1 "Treat as calibration reference"; OpenMPTBreakpointData1 "Open breakpoint data 1"; OpenADDBreakpointData1 "Open ADD breakpoint data 1"; BreakpointData2 "Breakpoint data for 2nd input (y-axis, column index):"; ReferenceBreakpointData2 "Treat as calibration reference"; OpenMPTBreakpointData2 "Open breakpoint data 2"; OpenADDBreakpointData2 "Open ADD breakpoint data 2"; IndexSearchMethod "Index search method:"; Table "Table data:"; ReferenceTable "Treat as calibration reference"; OpenMPTTable "Open table data"; OpenADDTable "Open ADD table data"; InterpMethod "Interpolation method:"; DisplayCalibrationNames "Block annotation with calibration data"; AdoptBlockName "Adopt block name from table name"; OutMin "Output minimum:"; OutMax "Output maximum:"; OutDataType "Output data type:"; IndexDataType "Index data type:"; FractionDataType "Fraction data type:"
      mask help:
      | Perform 2-D linear interpolation of input values using the specified table.
      | The first dimension corresponds to the top (or left) input.
      mask init:
      | % get and transmit data type from value
      | if strcmp(OutDataType,'Inherit: Inherit from data')
      |   val = Table;  nam = get_param(gcb,'Table');
      |   if evalin('base',['exist(''',nam,''',''var'')']),  s = evalin('base',nam);
      |     if isa(s,'mpt.Parameter') || isa(s,'Simulink.Parameter') || isa(s,'AVLmpt.Parameter')
      |       valDataType = s.DataType;
      |       if strcmp(valDataType,'auto'), valDataType = 'double'; end
      |     else
      |       valDataType = class(s);
      |     end
      |   else
      |       valDataType = class(val);
      |   end
      |   if strcmp(valDataType,'logical'), valDataType = 'boolean'; end
      |   set_param([gcb,'/Map'],'OutDataTypeStr',valDataType)
      | end
      | if 1
      |   val = BreakpointData1;  nam = get_param(gcb,'BreakpointData1');
      |   if evalin('base',['exist(''',nam,''',''var'')']),  s = evalin('base',nam);
      |     if isa(s,'mpt.Parameter') || isa(s,'Simulink.Parameter') || isa(s,'AVLmpt.Parameter')
      |       valDataType = s.DataType;
      |       if strcmp(valDataType,'auto'), valDataType = 'double'; end
      |     else
      |       valDataType = class(s);
      |     end
      |   else
      |       valDataType = class(val);
      |   end
      |   if strcmp(valDataType,'logical'), valDataType = 'boolean'; end
      |   set_param([gcb,'/u1'],'OutDataTypeStr',valDataType)
      | end
      | if 1
      |   val = BreakpointData2;  nam = get_param(gcb,'BreakpointData2');
      |   if evalin('base',['exist(''',nam,''',''var'')']),  s = evalin('base',nam);
      |     if isa(s,'mpt.Parameter') || isa(s,'Simulink.Parameter') || isa(s,'AVLmpt.Parameter')
      |       valDataType = s.DataType;
      |       if strcmp(valDataType,'auto'), valDataType = 'double'; end
      |     else
      |       valDataType = class(s);
      |     end
      |   else
      |       valDataType = class(val);
      |   end
      |   if strcmp(valDataType,'logical'), valDataType = 'boolean'; end
      |   set_param([gcb,'/u2'],'OutDataTypeStr',valDataType)
      | end
      | 
      | % © AVL S&F, C.A. Roduner, Nov/18/2009
      | if BlockConfiguration==1 && (~strcmp(get_param(gcb,'LinkStatus'),'resolved') ...
      |   || (~strncmp(get_param(gcb,'Referenceblock'),'AVLib',5) && ~exist('AVLib_Init','file') ) ), return, end
      | AVLib_Init( 'LookupTable2D_init', gcb, ...
      |   BlockConfiguration,IndexSearchMethod,InterpMethod, ...
      |   DisplayCalibrationNames,AdoptBlockName,  ...
      |   BreakpointData1,ReferenceBreakpointData1,OpenMPTBreakpointData1, OpenADDBreakpointData1, ...
      |   BreakpointData2,ReferenceBreakpointData2,OpenMPTBreakpointData2, OpenADDBreakpointData2, ...
      |   Table,ReferenceTable,OpenMPTTable,OpenADDTable, ...
      |   IndexDataType, FractionDataType, ...
      |   OutMin,OutMax,OutDataType ...
      | );
      mask Help: eval('try openDocu(gcb), catch try run([fileparts(which(''AVLib'')),''\..\AVLibDocu\openDocu'']), catch errordlg(''No documentation available on Matlab path.'',gcb,''modal''), end, end')
      mask TypeOptions BlockConfiguration: freeze | enable | default
      mask Callback BreakpointData1:
      | if strcmp(get_param(gcb,'BlockConfiguration'),'freeze'), return, end
      | AVLib_Init('Calibration_cb',gcb,'BreakpointData1')
      mask Callback OpenMPTBreakpointData1:
      | if strcmp(get_param(gcb,'BlockConfiguration'),'freeze'), return, end
      | AVLib_Init('OpenMPT_cb',gcb,'BreakpointData1')
      mask Callback OpenADDBreakpointData1:
      | if strcmp(get_param(gcb,'BlockConfiguration'),'freeze'), return, end
      | if strcmp(get_param(gcb,'OpenADDBreakpointData1'),'on')
      |   set_param(gcb,'OpenADDBreakpointData1','off')
      |   set_param(gcb,'BreakpointData1', connectADD(get_param(gcb,'BreakpointData1'),'axis1') )
      | end
      mask Callback BreakpointData2:
      | if strcmp(get_param(gcb,'BlockConfiguration'),'freeze'), return, end
      | AVLib_Init('Calibration_cb',gcb,'BreakpointData2')
      mask Callback OpenMPTBreakpointData2:
      | if strcmp(get_param(gcb,'BlockConfiguration'),'freeze'), return, end
      | AVLib_Init('OpenMPT_cb',gcb,'BreakpointData2')
      mask Callback OpenADDBreakpointData2:
      | if strcmp(get_param(gcb,'BlockConfiguration'),'freeze'), return, end
      | if strcmp(get_param(gcb,'OpenADDBreakpointData2'),'on')
      |   set_param(gcb,'OpenADDBreakpointData2','off')
      |   set_param(gcb,'BreakpointData2', connectADD(get_param(gcb,'BreakpointData2'),'axis2') )
      | end
      mask TypeOptions IndexSearchMethod: Evenly spaced points | Linear search | Binary search
      mask Callback Table:
      | if strcmp(get_param(gcb,'BlockConfiguration'),'freeze'), return, end
      | AVLib_Init('Calibration_cb',gcb,'Table')
      mask Callback OpenMPTTable:
      | if strcmp(get_param(gcb,'BlockConfiguration'),'freeze'), return, end
      | AVLib_Init('OpenMPT_cb',gcb,'Table')
      mask Callback OpenADDTable:
      | if strcmp(get_param(gcb,'BlockConfiguration'),'freeze'), return, end
      | if strcmp(get_param(gcb,'OpenADDTable'),'on')
      |   set_param(gcb,'OpenADDTable','off')
      |   set_param(gcb,'Table', connectADD(get_param(gcb,'Table'),'map') )
      | end
      mask TypeOptions InterpMethod: None - Flat | Linear
      mask Callback AdoptBlockName:
      | if strcmp(get_param(gcb,'BlockConfiguration'),'freeze'), return, end
      | AVLib_Init('AdoptBlockName_cb',gcb,get_param(gcb,'Table'))
      mask TypeOptions OutDataType: Inherit: Inherit from data | Inherit: Inherit via back propagation | double | single | int8 | uint8 | int16 | uint16 | int32 | uint32 | boolean
      mask TypeOptions IndexDataType: uint8 | uint16 | uint32
      mask TypeOptions FractionDataType: Inherit: Inherit via internal rule | double | single
      mask Display:
      | port_label('input',1,'x'), port_label('input',2,'y')
      | plot( getfield(get_param(gcb,'UserData'),'xy') )
      | plot( getfield(get_param(gcb,'UserData'),'xy_InterpMethod') )
      | color('blue'), plot( getfield(get_param(gcb,'UserData'),'xy_C') )
  Interpolation Using Prelookup : Interpolation_n-D  InternalRulePriority=Speed
      settings: CopyFcn=set_param(gcbh,'ShowName','off');
  OverRide : Subsystem  mask(override){}
      settings: CopyFcn=set_param(gcbh,'ShowName','off');
  OverRide_with_master_switch : Subsystem  mask(override){}
      settings: CopyFcn=set_param(gcbh,'ShowName','off');
  Parameter : Constant  Value=Parameter
      settings: CopyFcn=set_param(gcbh,'ShowName','off');
  Prelookup : PreLookup  BreakpointsData=[10:10:110]  ExtrapMethod=Linear
      settings: CopyFcn=set_param(gcbh,'ShowName','off');
  SwitchState : Relay  OnSwitchValue=SwitchOn_P  OffSwitchValue=SwitchOff_P
      settings: CopyFcn=set_param(gcbh,'ShowName','on');
      settings: AttributesFormatString=|
      | %<OnSwitchValue>
      | %<OffSwitchValue>
  n-D Lookup Table : Lookup_n-D  BreakpointsForDimension1=BreakpointData_One_A  BreakpointsForDimension2=BreakpointData_Two_A  Table=TableData_M  ExtrapMethod=Clip  UseLastTableValue=on  InternalRulePriority=Speed  RndMeth=Simplest  SaturateOnIntegerOverflow=on  InputSameDT=on
      settings: CopyFcn=set_param(gcbh,'ShowName','on');
  xbackground1 : Subsystem
      settings: CopyFcn=set_param(gcbh,'ShowName','off');
      mask Display: disp(' ')
  xbackground2 : Subsystem
      settings: CopyFcn=set_param(gcbh,'ShowName','off');
      mask Display: disp(' ')
  xbackground3 : Subsystem
      settings: CopyFcn=set_param(gcbh,'ShowName','off');
      mask Display: disp(' ')
  xbackground4 : Subsystem
      settings: CopyFcn=set_param(gcbh,'ShowName','off');
      mask Display: disp(' ')
